simulink model "four_CIFF_EM_sim_noise"  (R2020a)
settings: Solver=VariableStepAuto  StartTime=0.0  StopTime=1  MaxStep=1.55424749113179e-06  RelTol=0.0001
values from neighbouring files (symbols this model uses):
  a = [1 -1]    [CIC_Filter.m]    (also in Cascade_CIC_Filter.m; four_CIFF_EM.m = 0.9)
  Amax = 8    [four_CIFF_EM.m]
  Amp1 = 10*5.13e-6    (= 5.13e-05)    [four_CIFF_EM.m]
  b2 = 1    [four_CIFF_EM.m]
  C = 10e-12    (= 1e-11)    [four_CIFF_EM.m]
  finrad = Fin*2*pi    (= 188.495559215)    [four_CIFF_EM.m]
  g1 = 0.4    [four_CIFF_EM.m]
  g2 = 0.2    [four_CIFF_EM.m]
  g3 = 4    [four_CIFF_EM.m]
  g4 = 0.9    [four_CIFF_EM.m]
  g5 = 0.7    [four_CIFF_EM.m]
  GAIN = 50    [four_CIFF_EM.m]
  k = 1.38e-23    [four_CIFF_EM.m]
  Kcv = 4e12    (= 4000000000000)    [four_CIFF_EM.m]
  Kvf = 1.323e-4    (= 0.0001323)    [four_CIFF_EM.m]
  n = length(w)    [CIC_Filter.m]    (also in Cascade_CIC_Filter.m; Half_Band_Filter.m = 18; four_CIFF_EM.m = 0.08)
  noise1 = 10e-5    (= 0.0001)    [four_CIFF_EM.m]
  Ts = 1/Fs    (= 1.953125e-06)    [four_CIFF_EM.m]
  Vref = 1    [four_CIFF_EM.m]
  ws = sqrt(k/m)    [four_CIFF_EM.m]
undefined symbols (not defined in the file or in its folder): clock
libraries: SDtoolbox x8
settings Model: Creator=Chuqby  LastModifiedBy=Chuqby
settings DataIOCC: ReturnWorkspaceOutputs=off

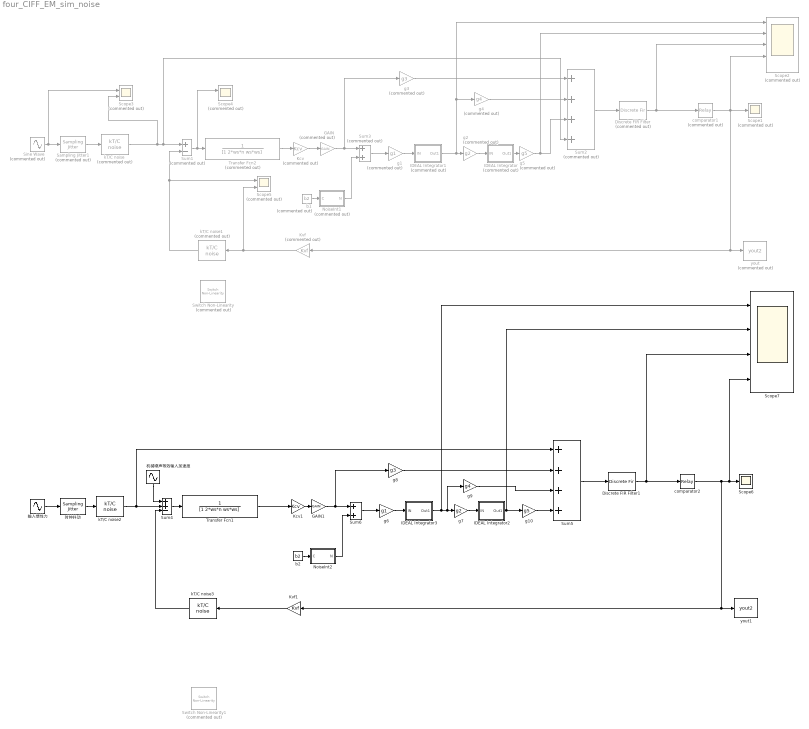
== system four_CIFF_EM_sim_noise ==
  Discrete FIR Filter : DiscreteFir  Commented=on  Coefficients=[1 -a]  SampleTime=Ts
  Discrete FIR Filter1 : DiscreteFir  Coefficients=[1 -a]  SampleTime=Ts
  GAIN : Gain  Commented=on  Gain=GAIN
  GAIN1 : Gain  Gain=GAIN
  IDEAL Integrator : Subsystem  Commented=on  mask(Integrator){Amax=Amax, Ts=Ts}
      mask prompts: Amax "Saturation"; Ts "Sample Time:"
      mask help:
      | Real discrete integrator with delay.
      | Models op-amp saturation and slew rate.
      mask Help:
      | Parameters:
      | Ts:       Sample time
      | G:         Finite op-amp gain (ideal op-amp G=1)
      | Amax:  Saturation value
      | sr:       slew rate in V/s
      mask Display: dpoly([0 1], [1 -1], 'z-')
  IDEAL Integrator1 : Subsystem  Commented=on  mask(Integrator){Amax=Amax, Ts=Ts}
      mask prompts: Amax "Saturation"; Ts "Sample Time:"
      mask help:
      | Real discrete integrator with delay.
      | Models op-amp saturation and slew rate.
      mask Help:
      | Parameters:
      | Ts:       Sample time
      | G:         Finite op-amp gain (ideal op-amp G=1)
      | Amax:  Saturation value
      | sr:       slew rate in V/s
      mask Display: dpoly([0 1], [1 -1], 'z-')
  IDEAL Integrator2 : Subsystem  mask(Integrator){Amax=Amax, Ts=Ts}
      mask prompts: Amax "Saturation"; Ts "Sample Time:"
      mask help:
      | Real discrete integrator with delay.
      | Models op-amp saturation and slew rate.
      mask Help:
      | Parameters:
      | Ts:       Sample time
      | G:         Finite op-amp gain (ideal op-amp G=1)
      | Amax:  Saturation value
      | sr:       slew rate in V/s
      mask Display: dpoly([0 1], [1 -1], 'z-')
  IDEAL Integrator3 : Subsystem  mask(Integrator){Amax=Amax, Ts=Ts}
      mask prompts: Amax "Saturation"; Ts "Sample Time:"
      mask help:
      | Real discrete integrator with delay.
      | Models op-amp saturation and slew rate.
      mask Help:
      | Parameters:
      | Ts:       Sample time
      | G:         Finite op-amp gain (ideal op-amp G=1)
      | Amax:  Saturation value
      | sr:       slew rate in V/s
      mask Display: dpoly([0 1], [1 -1], 'z-')
  Kcv : Gain  Commented=on  Gain=Kcv
  Kcv1 : Gain  Gain=Kcv
  Kvf : Gain  Commented=on  Gain=Kvf
  Kvf1 : Gain  Gain=Kvf
  NoiseInt1 : Subsystem  Commented=on  mask(OpAmp Noise){seed=sum(clock)^1/111, Ts=Ts, noise=noise1}
      mask prompts: seed "Random Number Seed:"; Ts "Sample Time:"; noise "Op-amp Noise Std. Dev.:"
      mask Display: disp('OpNoise')
  NoiseInt2 : Subsystem  mask(OpAmp Noise){seed=sum(clock)^1/111, Ts=Ts, noise=noise1}
      mask prompts: seed "Random Number Seed:"; Ts "Sample Time:"; noise "Op-amp Noise Std. Dev.:"
      mask Display: disp('OpNoise')
  Sampling Jitter1 : SDtoolbox/Sampling Jitter  Commented=on  Ts=Ts  delta=delta  seed=(sum(clock))^3.33
  Scope1 : Scope  Commented=on
  Scope2 : Scope  Commented=on  NumInputPorts=5
  Scope3 : Scope  Commented=on  NumInputPorts=2
  Scope4 : Scope  Commented=on  NumInputPorts=2
  Scope5 : Scope  Commented=on  NumInputPorts=2
  Scope6 : Scope
  Scope7 : Scope  NumInputPorts=4
  Sine Wave : Sin  Commented=on  Amplitude=Amp1  Frequency=finrad  SampleTime=0
  Sum1 : Sum  Commented=on  Inputs=+-
  Sum2 : Sum  Commented=on  Inputs=++++
  Sum3 : Sum  Commented=on
  Sum4 : Sum  Inputs=++-
  Sum5 : Sum  Inputs=++++
  Sum6 : Sum
  Switch Non-Linearity : SDtoolbox/Switch Non-Linearity  Commented=on  Ts=Ts  CS=Cs  VsupplyP=2  VsupplyN=-2  Size=20  KPN=175e-6  KPP=60e-6  VTN=0.5  VTP=-0.5  BS=0
  Switch Non-Linearity1 : SDtoolbox/Switch Non-Linearity  Commented=on  Ts=Ts  CS=Cs  VsupplyP=2  VsupplyN=-2  Size=20  KPN=175e-6  KPP=60e-6  VTN=0.5  VTP=-0.5  BS=0
  Transfer Fcn1 : TransferFcn  Denominator=[1 2*ws*n ws*ws]
  Transfer Fcn2 : TransferFcn  Commented=on  Denominator=[1 2*ws*n ws*ws]
  b1 : Constant  Commented=on  Value=b2
  b2 : Constant  Value=b2
  comparator1 : Relay  Commented=on  OnOutputValue=Vref  OffOutputValue=-Vref  ZeroCross=off
  comparator2 : Relay  OnOutputValue=Vref  OffOutputValue=-Vref  ZeroCross=off
  g1 : Gain  Commented=on  Gain=g1
  g10 : Gain  Gain=g5
  g2 : Gain  Commented=on  Gain=g2
  g3 : Gain  Commented=on  Gain=g3
  g4 : Gain  Commented=on  Gain=g4
  g5 : Gain  Commented=on  Gain=g5
  g6 : Gain  Gain=g1
  g7 : Gain  Gain=g2
  g8 : Gain  Gain=g3
  g9 : Gain  Gain=g4
  kT/C noise : SDtoolbox/kT//C noise  Commented=on  Ts=Ts  C=C  Temp=Temp  k=k  seed=floor(sum(clock))
  kT/C noise1 : SDtoolbox/kT//C noise  Commented=on  Ts=Ts  C=C  Temp=Temp  k=k  seed=floor(sum(clock))
  kT/C noise2 : SDtoolbox/kT//C noise  Ts=Ts  C=C  Temp=Temp  k=k  seed=floor(sum(clock))
  kT/C noise3 : SDtoolbox/kT//C noise  Ts=Ts  C=C  Temp=Temp  k=k  seed=floor(sum(clock))
  yout : ToWorkspace  Commented=on  VariableName=yout2  SampleTime=-1
      settings: Save2DSignal=2-D array (concatenate along first dimension)
  yout1 : ToWorkspace  VariableName=yout2  SampleTime=-1
      settings: Save2DSignal=2-D array (concatenate along first dimension)
  时钟抖动 : SDtoolbox/Sampling Jitter  Ts=Ts  delta=delta  seed=(sum(clock))^3.33
  机械噪声等效输入加速度 : Sin  Amplitude=3e-5  Frequency=finrad  SampleTime=0
  输入惯性力 : Sin  Amplitude=Amp1  Frequency=finrad  SampleTime=0
  wires:
  IDEAL Integrator1/1(Out1) -> g2/1, Scope2/1, g4/1
  g3/1 -> Sum2/1
  Sum1/1 -> Scope4/1, Transfer Fcn2/1
  Discrete FIR Filter/1 -> comparator1/1, Scope2/3
  g1/1 -> IDEAL Integrator1/1(IN)
  g2/1 -> IDEAL Integrator/1(IN)
  Sum2/1 -> Discrete FIR Filter/1
  GAIN/1 -> Sum3/1, g3/1
  Transfer Fcn2/1 -> Kcv/1
  Kcv/1 -> GAIN/1
  comparator1/1 -> Scope2/4, Scope1/1, yout/1, Kvf/1
  Sum3/1 -> g1/1
  Sine Wave/1 -> Sampling Jitter1/1, Scope3/1
  kT/C noise/1 -> Sum2/4, Sum1/1, Scope3/2
  Kvf/1 -> Scope5/2, kT/C noise1/1
  g4/1 -> Sum2/2
  NoiseInt1/1(N) -> Sum3/2
  b1/1 -> NoiseInt1/1(C)
  IDEAL Integrator/1(Out1) -> g5/1
  g5/1 -> Scope2/2, Sum2/3
  Sampling Jitter1/1 -> kT/C noise/1
  kT/C noise1/1 -> Scope5/1, Sum1/2
  Sum4/1 -> Transfer Fcn1/1
  时钟抖动/1 -> kT/C noise2/1
  g6/1 -> IDEAL Integrator3/1(IN)
  GAIN1/1 -> Sum6/1, g8/1
  Sum5/1 -> Discrete FIR Filter1/1
  NoiseInt2/1(N) -> Sum6/2
  Discrete FIR Filter1/1 -> Scope7/3, comparator2/1
  Kvf1/1 -> kT/C noise3/1
  b2/1 -> NoiseInt2/1(C)
  输入惯性力/1 -> 时钟抖动/1
  kT/C noise3/1 -> Sum4/3
  IDEAL Integrator3/1(Out1) -> Scope7/1, g7/1, g9/1
  g7/1 -> IDEAL Integrator2/1(IN)
  kT/C noise2/1 -> Sum5/1, Sum4/2
  Kcv1/1 -> GAIN1/1
  Sum6/1 -> g6/1
  g10/1 -> Sum5/4
  g9/1 -> Sum5/3
  g8/1 -> Sum5/2
  Transfer Fcn1/1 -> Kcv1/1
  机械噪声等效输入加速度/1 -> Sum4/1
  IDEAL Integrator2/1(Out1) -> Scope7/2, g10/1
  comparator2/1 -> Scope7/4, Scope6/1, yout1/1, Kvf1/1

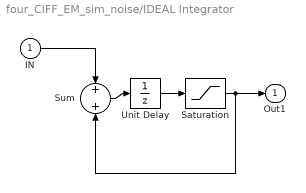
== system four_CIFF_EM_sim_noise/IDEAL Integrator ==
  IN : Inport
  Saturation : Saturate  UpperLimit=Amax  LowerLimit=-Amax
  Sum : Sum
  Unit Delay : UnitDelay  SampleTime=Ts
  Out1 : Outport
  wires:
  Sum/1 -> Unit Delay/1
  IN/1 -> Sum/1
  Unit Delay/1 -> Saturation/1
  Saturation/1 -> Out1/1, Sum/2

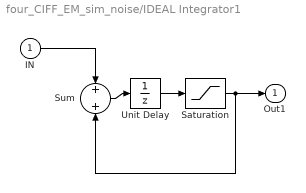
== system four_CIFF_EM_sim_noise/IDEAL Integrator1 ==
  IN : Inport
  Saturation : Saturate  UpperLimit=Amax  LowerLimit=-Amax
  Sum : Sum
  Unit Delay : UnitDelay  SampleTime=Ts
  Out1 : Outport
  wires:
  Sum/1 -> Unit Delay/1
  IN/1 -> Sum/1
  Unit Delay/1 -> Saturation/1
  Saturation/1 -> Out1/1, Sum/2

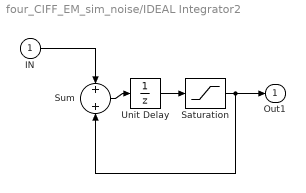
== system four_CIFF_EM_sim_noise/IDEAL Integrator2 ==
  IN : Inport
  Saturation : Saturate  UpperLimit=Amax  LowerLimit=-Amax
  Sum : Sum
  Unit Delay : UnitDelay  SampleTime=Ts
  Out1 : Outport
  wires:
  Sum/1 -> Unit Delay/1
  IN/1 -> Sum/1
  Unit Delay/1 -> Saturation/1
  Saturation/1 -> Out1/1, Sum/2

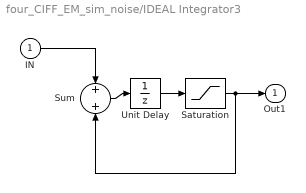
== system four_CIFF_EM_sim_noise/IDEAL Integrator3 ==
  IN : Inport
  Saturation : Saturate  UpperLimit=Amax  LowerLimit=-Amax
  Sum : Sum
  Unit Delay : UnitDelay  SampleTime=Ts
  Out1 : Outport
  wires:
  Sum/1 -> Unit Delay/1
  IN/1 -> Sum/1
  Unit Delay/1 -> Saturation/1
  Saturation/1 -> Out1/1, Sum/2

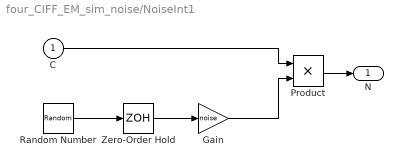
== system four_CIFF_EM_sim_noise/NoiseInt1 ==
  C : Inport
  Gain : Gain  Gain=noise
  Product : Product
  Random Number : RandomNumber  Seed=seed  SampleTime=Ts
  Zero-Order Hold : ZeroOrderHold  SampleTime=Ts
  N : Outport  InitialOutput=0
  wires:
  Random Number/1 -> Zero-Order Hold/1
  Zero-Order Hold/1 -> Gain/1
  Product/1 -> N/1
  Gain/1 -> Product/2
  C/1 -> Product/1

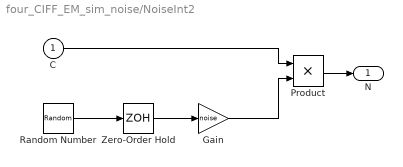
== system four_CIFF_EM_sim_noise/NoiseInt2 ==
  C : Inport
  Gain : Gain  Gain=noise
  Product : Product
  Random Number : RandomNumber  Seed=seed  SampleTime=Ts
  Zero-Order Hold : ZeroOrderHold  SampleTime=Ts
  N : Outport  InitialOutput=0
  wires:
  Random Number/1 -> Zero-Order Hold/1
  Zero-Order Hold/1 -> Gain/1
  Product/1 -> N/1
  Gain/1 -> Product/2
  C/1 -> Product/1
